simulink model "single_phase_cycloconverter"  (Simulink 6.1)
settings: Solver=ode23tb  StartTime=0.0  StopTime=0.2  MaxStep=1e-4  RelTol=1e-3  AbsTol=.01
libraries: powerlib x12, powerlib_extras x2
settings Model: LastModifiedBy=ThinkPad
settings DebuggingCC: SolverPrmCheckMsg=warning

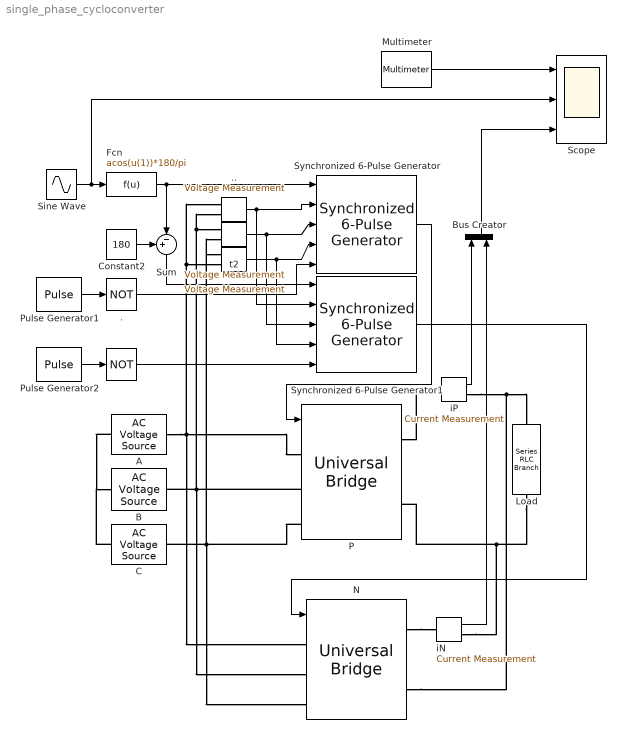
== system single_phase_cycloconverter ==
  " " : Logic  Operator=NOT  AllPortsSameDT=off  OutDataTypeMode=Boolean
  "   " : powerlib/Measurements/Voltage Measurement  PhasorSimulation=off  OutputType=Complex  PSBequivalent=0
  " ." : Logic  Operator=NOT  AllPortsSameDT=off  OutDataTypeMode=Boolean
  " .." : powerlib/Measurements/Voltage Measurement  PhasorSimulation=off  OutputType=Complex  PSBequivalent=0
  A : powerlib/Electrical Sources/AC Voltage Source  Amplitude=100  Phase=30  Frequency=50  SampleTime=0  Measurements=None
  B : powerlib/Electrical Sources/AC Voltage Source  Amplitude=100  Phase=-90  Frequency=50  SampleTime=0  Measurements=None
  Bus Creator : BusCreator  Orientation=up  DialogController=Simulink.DDGSource_Bus  Inputs=2
  C : powerlib/Electrical Sources/AC Voltage Source  Amplitude=100  Phase=-210  Frequency=50  SampleTime=0  Measurements=None
  Constant2 : Constant  Value=180
  Fcn : Fcn  Expr=acos(u(1))*180/pi
  Load : powerlib/Elements/Series RLC Branch  Orientation=down  PhysicalDomain=powersysdomain  SubClassName=unknown  LeftPortType=p1  RightPortType=p1  LConnTagsString=__new0  RConnTagsString=__new0  Resistance=1  Inductance=0.01  Capacitance=inf  Measurements=Branch voltage and current
  Multimeter : powerlib/Measurements/Multimeter  Tag=PoWeRsYsTeMmEaSuReMeNt  PhasorSimulation=off  OutputType=Magnitude  sel=[1 2]  L=2  Gain=[1 1]  yselected={'Ub: Load','Ib: Load'};  PSBOutputType=1  PSBequivalent=0  AxesSetting=[0,0.1,-100,100]  Display=0  SavedBlockNames=-11
      settings: AttributesFormatString=\n
  N : powerlib/Power Electronics/Universal Bridge  Arms=3  SnubberResistance=1e5  SnubberCapacitance=inf  Device=Thyristors  Ron=1e-3  Lon=0  ForwardVoltages="[  0  0  ]"  ForwardVoltage=0  GTOparameters=[ 10e-6 , 20e-6 ]  IGBTparameters=[ 1e-6 , 2e-6 ]  Measurements=None
  P : powerlib/Power Electronics/Universal Bridge  Arms=3  SnubberResistance=1e5  SnubberCapacitance=inf  Device=Thyristors  Ron=1e-3  Lon=0  ForwardVoltages="[  0  0  ]"  ForwardVoltage=0  GTOparameters=[ 10e-6 , 20e-6 ]  IGBTparameters=[ 1e-6 , 2e-6 ]  Measurements=None
  Pulse Generator1 : DiscretePulseGenerator  PulseType=Time based  Period=0.1  PulseWidth=48  PhaseDelay=0.01
  Pulse Generator2 : DiscretePulseGenerator  PulseType=Time based  Period=0.1  PulseWidth=48  PhaseDelay=0.06
  Scope : Scope  NumInputPorts=3
      settings: TimeRange=0.2  YMin=-200~-1~-50  YMax=200~1~150  Decimation=5  SampleInput=on  SampleTime=1e-4
  Sine Wave : Sin  Amplitude=0.8  Frequency=62.8  SampleTime=0
  Sum : Sum  Orientation=down  Inputs=+-|
  Synchronized 6-Pulse Generator : powerlib_extras/Control  Blocks/Synchronized 6-Pulse Generator  freq=50  pwidth=10  Double_Pulse=on
  Synchronized 6-Pulse Generator1 : powerlib_extras/Control  Blocks/Synchronized 6-Pulse Generator  freq=50  pwidth=10  Double_Pulse=on
  iN : powerlib/Measurements/Current Measurement  PhasorSimulation=off  OutputType=Complex  PSBequivalent=0
  iP : powerlib/Measurements/Current Measurement  PhasorSimulation=off  OutputType=Complex  PSBequivalent=0
  t2 : powerlib/Measurements/Voltage Measurement  PhasorSimulation=off  OutputType=Complex  PSBequivalent=0
  wires:
  " .."/1 -> Synchronized 6-Pulse Generator/2, Synchronized 6-Pulse Generator1/2
  t2/1 -> Synchronized 6-Pulse Generator/3, Synchronized 6-Pulse Generator1/3
  "   "/1 -> Synchronized 6-Pulse Generator/4, Synchronized 6-Pulse Generator1/4
  Fcn/1 -> Sum/2, Synchronized 6-Pulse Generator/1
  Multimeter/1 -> Scope/1
  Synchronized 6-Pulse Generator1/1 -> N/1
  Sine Wave/1 -> Fcn/1, Scope/2
  Synchronized 6-Pulse Generator/1 -> P/1
  Constant2/1 -> Sum/1
  Sum/1 -> Synchronized 6-Pulse Generator1/1
  iP/1 -> Bus Creator/1
  iN/1 -> Bus Creator/2
  Bus Creator/1 -> Scope/3
  Pulse Generator1/1 -> " ."/1
  " ."/1 -> Synchronized 6-Pulse Generator/5
  Pulse Generator2/1 -> " "/1
  " "/1 -> Synchronized 6-Pulse Generator1/5
  connections:
  A/LConn1 -- C/LConn1 -- B/LConn1
  P/LConn3 -- C/RConn1 -- N/LConn3 -- t2/LConn2 -- "   "/LConn1
  P/LConn2 -- B/RConn1 -- N/LConn2 -- " .."/LConn2 -- t2/LConn1
  Load/RConn1 -- P/RConn2 -- iN/RConn1
  A/RConn1 -- P/LConn1 -- N/LConn1 -- " .."/LConn1 -- "   "/LConn2
  iP/RConn1 -- Load/LConn1 -- N/RConn2
  P/RConn1 -- iP/LConn1
  N/RConn1 -- iN/LConn1
